simulink model "BLDCmotorControl_FOC_R2017b_fixdt"  (R2017b)
settings: Solver=FixedStepDiscrete  StartTime=0  StopTime=0.5  FixedStep=Ts  MaxStep=1e-6  RelTol=1e-6  AbsTol=1e-6  EnableMultiTasking=on
PreLoadFcn:
  | addpath(pwd);
  | addpath(genpath('01_Libraries'));
  | addpath(genpath('02_Figures'));
  | addpath(genpath('03_CreateParamTable'));
InitFcn:
  | init_model;
values from neighbouring files (symbols this model uses):
  a_elecAngle = 60    [init_model.m]
  b_diagEna = 1    [init_model.m]
  b_fieldWeakEna = 0    [init_model.m]
  b_selPhaABCurrMeas = 1    [init_model.m]
  cf_currFilt = 0.12    [init_model.m]
  cf_idKb = 1000 * Ts_ctrl    (= 0.06)    [init_model.m]
  cf_idKi = 100 * Ts_ctrl    (= 0.006)    [init_model.m]
  cf_idKp = 1    [init_model.m]
  cf_iqKb = 1000 * Ts_ctrl    (= 0.06)    [init_model.m]
  cf_iqKi = 100 * Ts_ctrl    (= 0.006)    [init_model.m]
  cf_iqKiLimProt = 40.7 * Ts_ctrl    (= 0.002442)    [init_model.m]
  cf_iqKp = 0.5    [init_model.m]
  cf_iqKpLimProt = 7.2    [init_model.m]
  cf_nKb = 1000 * Ts_ctrl    (= 0.06)    [init_model.m]
  cf_nKi = 20.4 * Ts_ctrl    (= 0.001224)    [init_model.m]
  cf_nKp = 1.18    [init_model.m]
  cf_nKpLimProt = 5    [init_model.m]
  cf_speedCoef = round(f_ctrl * a_mechAngle * (pi/180) * (30/pi))    [init_model.m]
  CTRL_COM = 0    [init_model.m]
  dV_openRate = 1000 * Ts_ctrl    (= 0.06)    [init_model.m]
  dz_cntTrnsDetHi = 40    [init_model.m]
  dz_cntTrnsDetLo = 20    [init_model.m]
  i_max = i_max * i_sca    (= 750)    [init_model.m]
  id_fieldWeak_M1 = [  0   0  0.05  0.25    1    2    3    4  4.5  4.8   5   5] * i_sca    [init_model.m]
  iq_max_M1 = sqrt(i_max^2 - iq_max_XA.^2)    [init_model.m]
  n_commAcvLo = 15    [init_model.m]
  n_commDeacvHi = 30    [init_model.m]
  n_max = 800    [init_model.m]
  n_stdStillDet = 3    [init_model.m]
  OPEN_MODE = 0    [init_model.m]
  r_cos_M1 = cos((a_elecAngle_XA + 30)*(pi/180))    [init_model.m]
  r_errInpTgtThres = 200    [init_model.m]
  r_sin_M1 = sin((a_elecAngle_XA + 30)*(pi/180))    [init_model.m]
  r_whl = 6.5 * 2.54 * 1e-2 / 2    (= 0.08255)    [init_model.m]
  SPD_MODE = 2    [init_model.m]
  t_errDequal = 2.0 * f_ctrl    (= 32000)    [init_model.m]
  t_errQual = 0.6 * f_ctrl    (= 9600)    [init_model.m]
  TRQ_MODE = 3    [init_model.m]
  Ts = 5e-6    (= 5e-06)    [init_model.m]
  Ts_ctrl = 6e-5    (= 6e-05)    [init_model.m]
  Vd_max = 1000 - V_margin    (= 900)    [init_model.m]
  vec_hallToPos = [0 2 0 1 4 3 5 0]    [init_model.m]
  VLT_MODE = 1    [init_model.m]
  Vq_max_M1 = sqrt(Vd_max^2 - Vq_max_XA.^2)    [init_model.m]
  z_commutMap_M1 = [-1 -1  0  1  1  0 ... (first row only)    [init_model.m]
  z_ctrlModReq = 1    [init_model.m]
  z_ctrlTypSel = 1    [init_model.m]
  z_maxCntRst = 2000    [init_model.m]
undefined symbols (not defined in the file or in its folder): DiscIntNeverNeededParam, sigbuilder_block, V_max, V_min
libraries: BLDC_controller_Lib x11, simulink x11, powerlib x6, pePwmGenerator x1
(part 3 of 3)

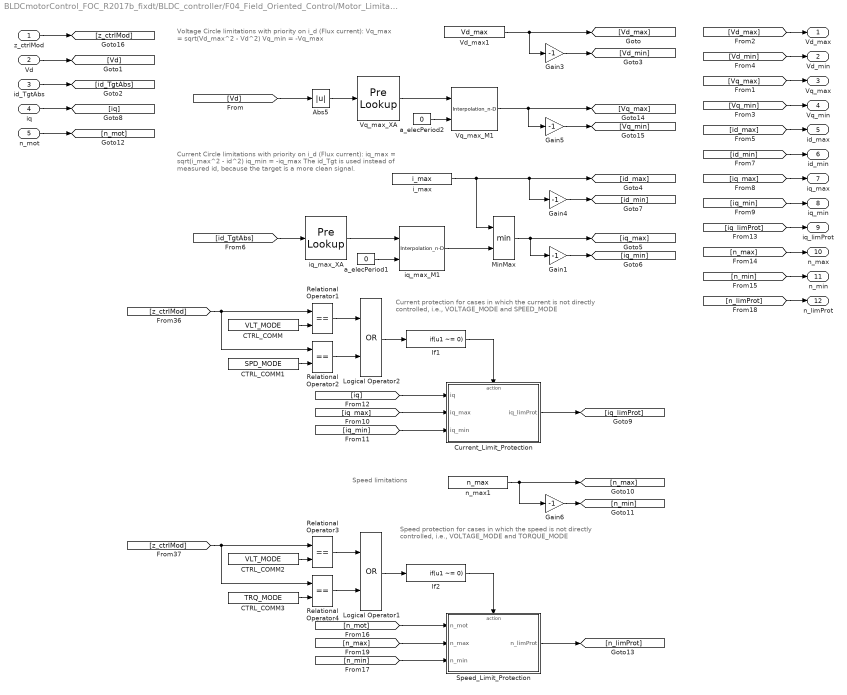
== system BLDCmotorControl_FOC_R2017b_fixdt/BLDC_controller/F04_Field_Oriented_Control/Motor_Limitations ==
  note: Voltage Circle limitations with priority on i_d (Flux current):
      | Vq_max = sqrt(Vd_max^2 - Vd^2)
      | Vq_min = -Vq_max
  note: Current Circle limitations with priority on i_d (Flux current):
      | iq_max = sqrt(i_max^2 - id^2)
      | iq_min = -iq_max
      |
      | The id_Tgt is used instead of measured id, because the target is a more clean signal.
  note: Speed limitations
  note: Current protection
      | for cases in which the current is not directly controlled, i.e., VOLTAGE_MODE and SPEED_MODE
  note: Speed protection
      | for cases in which the speed is not directly controlled, i.e., VOLTAGE_MODE and TORQUE_MODE
  z_ctrlMod : Inport
  Vd : Inport  Port=2
  id_TgtAbs : Inport  Port=3
  iq : Inport  Port=4
  n_mot : Inport  Port=5
  Abs5 : Abs  OutDataTypeStr=Inherit: Inherit via back propagation  RndMeth=Zero
  CTRL_COMM : Constant  Value=VLT_MODE  OutDataTypeStr=Inherit: Inherit via back propagation
  CTRL_COMM1 : Constant  Value=SPD_MODE  OutDataTypeStr=Inherit: Inherit via back propagation
  CTRL_COMM2 : Constant  Value=VLT_MODE  OutDataTypeStr=Inherit: Inherit via back propagation
  CTRL_COMM3 : Constant  Value=TRQ_MODE  OutDataTypeStr=Inherit: Inherit via back propagation
  Current_Limit_Protection : Subsystem
  Gain{1,3..6} (5 alike) : Gain  Tag=struct('comment',struct('text','','placement',1),'logdata',struct('maxnumvals',inf,'plotchannels',[],'loggingmode',3,'channels',1),'output',struct('variable','','description','','name','$S_$B','width',1,'address','','max',NaN,'min',NaN,'class','default','type','CONTINUOUS','scaling','','lsb',1,'offset',0,'arb',0,'freeze',1,'unit','','autoscalingmode',1,'lowerheadroom',1,'upperheadroom',1,'headroomunit','bit','keepdatatype',1,'checkmin',0,'checkmax',0,'castoutput',0,'show',0),'gain',struct('variable','','description','','name','$S_$B_gain','width',1,'address','','max',NaN,'min',NaN,'class','default','type','CONTINUOUS','scaling','','lsb',1,'offset',0,'arb',0,'freeze',1,'unit','','keepdatatype',1,'value','1','scalar',0,'tolerance',1),'scalingvalid',0,'date',730486)  Gain=-1  RndMeth=Zero  OutDataTypeStr=Inherit: Same as input  ParamDataTypeStr=Inherit: Same as input
  If1 : If  IfExpression=u1 ~= 0  ShowElse=off
  If2 : If  IfExpression=u1 ~= 0  ShowElse=off
  Logical Operator1 : Logic  Operator=OR  AllPortsSameDT=off  OutDataTypeStr=boolean
  Logical Operator2 : Logic  Operator=OR  AllPortsSameDT=off  OutDataTypeStr=boolean
  MinMax : MinMax  Inputs=2
  Relational Operator{1..4} (4 alike) : RelationalOperator  Operator===  OutDataTypeStr=boolean  RndMeth=Simplest
  Speed_Limit_Protection : Subsystem
  Vd_max1 : Constant  Value=Vd_max  OutDataTypeStr=fixdt(1,16,4)
  Vq_max_M1 : Interpolation_n-D  NumberOfTableDimensions=1  Table=Vq_max_M1  InterpMethod=Flat  ExtrapMethod=Clip  ValidIndexMayReachLast=on  OutDataTypeStr=fixdt(1,16,4)  InternalRulePriority=Speed  RndMeth=Simplest
      settings: InputPortMap=u0,u1
  Vq_max_XA : PreLookup  BreakpointsData=Vq_max_XA  OutputSelection=Index only  IndexSearchMethod=Evenly spaced points  BeginIndexSearchUsingPreviousIndexResult=on  IndexDataTypeStr=uint8  FractionDataTypeStr=fixdt(0,8,6)  RndMeth=Simplest
  a_elecPeriod1 : Constant  Value=0  OutDataTypeStr=uint8
  a_elecPeriod2 : Constant  Value=0  OutDataTypeStr=uint8
  i_max : Constant  Value=i_max  OutDataTypeStr=fixdt(1,16,4)
  iq_max_M1 : Interpolation_n-D  NumberOfTableDimensions=1  Table=iq_max_M1  InterpMethod=Flat  ExtrapMethod=Clip  ValidIndexMayReachLast=on  OutDataTypeStr=fixdt(1,16,4)  InternalRulePriority=Speed  RndMeth=Simplest
      settings: InputPortMap=u0,u1
  iq_max_XA : PreLookup  BreakpointsData=iq_max_XA  OutputSelection=Index only  IndexSearchMethod=Evenly spaced points  BeginIndexSearchUsingPreviousIndexResult=on  IndexDataTypeStr=uint8  FractionDataTypeStr=fixdt(0,8,6)  RndMeth=Simplest
  n_max1 : Constant  Value=n_max  OutDataTypeStr=fixdt(1,16,4)
  Vd_max : Outport  OutputWhenDisabled=reset  InitialOutput=V_max
  Vd_min : Outport  Port=2  OutputWhenDisabled=reset  InitialOutput=V_min
  Vq_max : Outport  Port=3  OutputWhenDisabled=reset  InitialOutput=V_max
  Vq_min : Outport  Port=4  OutputWhenDisabled=reset  InitialOutput=V_min
  id_max : Outport  Port=5  OutputWhenDisabled=reset  InitialOutput=V_max
  id_min : Outport  Port=6  OutputWhenDisabled=reset  InitialOutput=V_min
  iq_max : Outport  Port=7  OutputWhenDisabled=reset  InitialOutput=V_max
  iq_min : Outport  Port=8  OutputWhenDisabled=reset  InitialOutput=V_min
  iq_limProt : Outport  Port=9  OutputWhenDisabled=reset  InitialOutput=V_min
  n_max : Outport  Port=10  OutputWhenDisabled=reset  InitialOutput=V_max
  n_min : Outport  Port=11  OutputWhenDisabled=reset  InitialOutput=V_min
  n_limProt : Outport  Port=12  OutputWhenDisabled=reset  InitialOutput=V_min
  wires:
  Vq_max_XA/1 -> Vq_max_M1/1
  [Vq_min] -> Vq_min/1
  [Vq_max] -> Vq_max/1
  Gain5/1 -> [Vq_min]
  Vd_max1/1 -> Gain3/1, [Vd_max]
  [Vd] -> Abs5/1
  Vd/1 -> [Vd]
  id_TgtAbs/1 -> [id_TgtAbs]
  [Vd_max] -> Vd_max/1
  [Vd_min] -> Vd_min/1
  Gain3/1 -> [Vd_min]
  Gain4/1 -> [id_min]
  i_max/1 -> MinMax/1, Gain4/1, [id_max]
  [id_TgtAbs] -> iq_max_XA/1
  MinMax/1 -> [iq_max], Gain1/1
  Gain1/1 -> [iq_min]
  iq_max_XA/1 -> iq_max_M1/1
  [id_min] -> id_min/1
  [id_max] -> id_max/1
  [iq_max] -> iq_max/1
  [iq_min] -> iq_min/1
  iq/1 -> [iq]
  [iq_limProt] -> iq_limProt/1
  n_max1/1 -> [n_max], Gain6/1
  Gain6/1 -> [n_min]
  [n_min] -> n_min/1
  [n_max] -> n_max/1
  n_mot/1 -> [n_mot]
  [n_limProt] -> n_limProt/1
  z_ctrlMod/1 -> [z_ctrlMod]
  Relational Operator1/1 -> Logical Operator2/1
  [z_ctrlMod] -> Relational Operator2/1, Relational Operator1/1
  Logical Operator2/1 -> If1/1
  Relational Operator2/1 -> Logical Operator2/2
  CTRL_COMM/1 -> Relational Operator1/2
  CTRL_COMM1/1 -> Relational Operator2/2
  CTRL_COMM3/1 -> Relational Operator4/2
  CTRL_COMM2/1 -> Relational Operator3/2
  Relational Operator4/1 -> Logical Operator1/2
  Logical Operator1/1 -> If2/1
  [z_ctrlMod] -> Relational Operator3/1, Relational Operator4/1
  Relational Operator3/1 -> Logical Operator1/1
  [iq_max] -> Current_Limit_Protection/2(iq_max)
  [iq] -> Current_Limit_Protection/1(iq)
  [iq_min] -> Current_Limit_Protection/3(iq_min)
  Current_Limit_Protection/1(iq_limProt) -> [iq_limProt]
  [n_max] -> Speed_Limit_Protection/2(n_max)
  [n_mot] -> Speed_Limit_Protection/1(n_mot)
  [n_min] -> Speed_Limit_Protection/3(n_min)
  Speed_Limit_Protection/1(n_limProt) -> [n_limProt]
  If1/1 -> Current_Limit_Protection/Action
  If2/1 -> Speed_Limit_Protection/Action
  iq_max_M1/1 -> MinMax/2
  a_elecPeriod1/1 -> iq_max_M1/2
  Vq_max_M1/1 -> Gain5/1, [Vq_max]
  a_elecPeriod2/1 -> Vq_max_M1/2
  Abs5/1 -> Vq_max_XA/1

== system BLDCmotorControl_FOC_R2017b_fixdt/BLDC_controller/F04_Field_Oriented_Control/Open_Mode ==
  note: This will reduce the control command to 0 with a predefined rate.
  Vq_prev : Inport
  Action Port : ActionPort  InitializeStates=reset  ActionType=default
  Constant23 : Constant  Value=0  OutDataTypeStr=Inherit: Inherit via back propagation
  Data Type Conversion : DataTypeConversion  OutDataTypeStr=fixdt(1,28,16)
  Data Type Conversion1 : DataTypeConversion  OutDataTypeStr=fixdt(1,16,4)
  Gain3 : Gain  Tag=struct('comment',struct('text','','placement',1),'logdata',struct('maxnumvals',inf,'plotchannels',[],'loggingmode',3,'channels',1),'output',struct('variable','','description','','name','$S_$B','width',1,'address','','max',NaN,'min',NaN,'class','default','type','CONTINUOUS','scaling','','lsb',1,'offset',0,'arb',0,'freeze',1,'unit','','autoscalingmode',1,'lowerheadroom',1,'upperheadroom',1,'headroomunit','bit','keepdatatype',1,'checkmin',0,'checkmax',0,'castoutput',0,'show',0),'gain',struct('variable','','description','','name','$S_$B_gain','width',1,'address','','max',NaN,'min',NaN,'class','default','type','CONTINUOUS','scaling','','lsb',1,'offset',0,'arb',0,'freeze',1,'unit','','keepdatatype',1,'value','1','scalar',0,'tolerance',1),'scalingvalid',0,'date',730486)  Gain=-1  RndMeth=Zero  OutDataTypeStr=Inherit: Same as input
  Rate_Limiter : BLDC_controller_Lib/Rate_Limiter  SystemSampleTime=-1
  dV_openRate : Constant  Value=dV_openRate  OutDataTypeStr=fixdt(1,28,16)
  rising_edge_init : BLDC_controller_Lib/rising_edge_init
  Vq_Open : Outport
  wires:
  Vq_prev/1 -> [Vq_prev]
  Constant23/1 -> Rate_Limiter/1
  rising_edge_init/1 -> Rate_Limiter/3
  Gain3/1 -> Rate_Limiter/5
  dV_openRate/1 -> Gain3/1, Rate_Limiter/4
  Data Type Conversion1/1 -> [Vq_Open]
  [Vq_Open] -> Vq_Open/1
  Rate_Limiter/1 -> Data Type Conversion1/1
  [Vq_prev] -> Data Type Conversion/1
  Data Type Conversion/1 -> Rate_Limiter/2

== system BLDCmotorControl_FOC_R2017b_fixdt/BLDC_controller/F04_Field_Oriented_Control/Park_Transform ==
  note: Park Transform:
      | iq = -i_alpha*sin(angle) + i_beta*cos(angle)
      | id = i_alpha*cos(angle) + i_beta*sin(angle)
  i_apha : Inport
  i_beta : Inport  Port=2
  r_sin : Inport  Port=3
  r_cos : Inport  Port=4
  Divide{1..4} (4 alike) : Product  Inputs=**  RndMeth=Simplest  OutDataTypeStr=Inherit: Same as first input
  Sum1 : Sum  OutDataTypeStr=fixdt(1,16,4)  RndMeth=Simplest  SaturateOnIntegerOverflow=on
  Sum6 : Sum  Inputs=-+  OutDataTypeStr=fixdt(1,16,4)  RndMeth=Simplest  SaturateOnIntegerOverflow=on
  iq_Raw : Outport
  id_Raw : Outport  Port=2
  wires:
  r_sin/1 -> [r_sin]
  i_beta/1 -> [i_beta]
  i_apha/1 -> [i_apha]
  r_cos/1 -> [r_cos]
  [r_sin] -> Divide4/2
  [i_apha] -> Divide4/1
  Divide4/1 -> Sum6/1
  Divide1/1 -> Sum6/2
  [i_beta] -> Divide1/1
  [r_cos] -> Divide1/2
  Sum6/1 -> iq_Raw/1
  Divide2/1 -> Sum1/1
  [i_apha] -> Divide2/1
  [r_cos] -> Divide2/2
  Divide3/1 -> Sum1/2
  [i_beta] -> Divide3/1
  [r_sin] -> Divide3/2
  Sum1/1 -> id_Raw/1

== system BLDCmotorControl_FOC_R2017b_fixdt/BLDC_controller/F04_Field_Oriented_Control/Speed_Mode ==
  note: This product is necessary because the value is an input to the Integral part of the PI controller
  r_inpTgtSca : Inport
  Vq_max : Inport  Port=2
  Vq_min : Inport  Port=3
  n_mot : Inport  Port=4
  n_max : Inport  Port=5
  n_min : Inport  Port=6
  iq_limProt : Inport  Port=7
  Action Port : ActionPort  InitializeStates=reset  ActionType=case
  Divide1 : Product  Inputs=**  OutDataTypeStr=fixdt(1,16,10)  RndMeth=Simplest
  PI_backCalc_fixdt_n : BLDC_controller_Lib/PI_backCalc_fixdt  SystemSampleTime=-1
  Saturation Dynamic1 : simulink/Discontinuities/Saturation Dynamic  OutMin=[]  OutMax=[]  OutDataTypeStr=Inherit: Same as second input  OutDataType=fixdt(1, 16)  OutScaling=2^-10  DoSatur=off
  Signal Conversion2 : SignalConversion  OverrideOpt=off
  Sum3 : Sum  Inputs=|+-  RndMeth=Simplest  SaturateOnIntegerOverflow=on
  cf_iqKiLimProt : Constant  Value=cf_iqKiLimProt  OutDataTypeStr=fixdt(0,16,16)
  cf_nKb : Constant  Value=cf_nKb  OutDataTypeStr=fixdt(0,16,16)
  cf_nKi : Constant  Value=cf_nKi  VectorParams1D=off  OutDataTypeStr=fixdt(0,16,16)
  cf_nKp : Constant  Value=cf_nKp  OutDataTypeStr=fixdt(0,16,8)
  Vq_Spd : Outport
  wires:
  [Vq_min] -> PI_backCalc_fixdt_n/7
  [Vq_max] -> PI_backCalc_fixdt_n/6
  cf_nKi/1 -> PI_backCalc_fixdt_n/3
  cf_nKb/1 -> PI_backCalc_fixdt_n/4
  cf_nKp/1 -> PI_backCalc_fixdt_n/2
  [n_mot] -> Sum3/2
  Sum3/1 -> PI_backCalc_fixdt_n/1
  r_inpTgtSca/1 -> [r_inpTgtSca]
  Vq_max/1 -> [Vq_max]
  Vq_min/1 -> [Vq_min]
  n_mot/1 -> [n_mot]
  [n_min] -> Saturation Dynamic1/3
  [n_max] -> Saturation Dynamic1/1
  [r_inpTgtSca] -> Saturation Dynamic1/2
  Saturation Dynamic1/1 -> Sum3/1
  n_min/1 -> [n_min]
  n_max/1 -> [n_max]
  PI_backCalc_fixdt_n/1 -> Signal Conversion2/1
  iq_limProt/1 -> [iq_limProt]
  Divide1/1 -> PI_backCalc_fixdt_n/5
  cf_iqKiLimProt/1 -> Divide1/2
  [iq_limProt] -> Divide1/1
  Signal Conversion2/1 -> Vq_Spd/1

== system BLDCmotorControl_FOC_R2017b_fixdt/BLDC_controller/F04_Field_Oriented_Control/Torque_Mode ==
  r_inpTgtSca : Inport
  Vq_max : Inport  Port=2
  Vq_min : Inport  Port=3
  iq : Inport  Port=4
  iq_max : Inport  Port=5
  iq_min : Inport  Port=6
  n_limProt : Inport  Port=7
  Action Port : ActionPort  InitializeStates=reset  ActionType=case
  PI_backCalc_fixdt_Iq : BLDC_controller_Lib/PI_backCalc_fixdt  SystemSampleTime=-1
  Saturation Dynamic : simulink/Discontinuities/Saturation Dynamic  OutMin=[]  OutMax=[]  OutDataTypeStr=Inherit: Same as second input  OutDataType=fixdt(1, 16)  OutScaling=2^-10  DoSatur=off
  Signal Conversion2 : SignalConversion  OverrideOpt=off
  Sum1 : Sum  Inputs=|+-  RndMeth=Simplest  SaturateOnIntegerOverflow=on
  Sum2 : Sum  RndMeth=Simplest  SaturateOnIntegerOverflow=on
  cf_iqKb : Constant  Value=cf_iqKb  OutDataTypeStr=fixdt(0,16,16)
  cf_iqKi : Constant  Value=cf_iqKi  OutDataTypeStr=fixdt(0,16,16)
  cf_iqKp : Constant  Value=cf_iqKp  OutDataTypeStr=fixdt(0,16,8)
  constant : Constant  Value=0  OutDataTypeStr=Inherit: Inherit via back propagation
  Vq_Trq : Outport
  wires:
  cf_iqKi/1 -> PI_backCalc_fixdt_Iq/3
  [r_inpTgtSca] -> Sum2/1
  [Vq_max] -> PI_backCalc_fixdt_Iq/6
  [Vq_min] -> PI_backCalc_fixdt_Iq/7
  [iq] -> Sum1/2
  Sum1/1 -> PI_backCalc_fixdt_Iq/1
  cf_iqKb/1 -> PI_backCalc_fixdt_Iq/4
  cf_iqKp/1 -> PI_backCalc_fixdt_Iq/2
  Vq_max/1 -> [Vq_max]
  r_inpTgtSca/1 -> [r_inpTgtSca]
  Vq_min/1 -> [Vq_min]
  iq/1 -> [iq]
  PI_backCalc_fixdt_Iq/1 -> Signal Conversion2/1
  iq_min/1 -> [iq_min]
  iq_max/1 -> [iq_max]
  [iq_min] -> Saturation Dynamic/3
  [iq_max] -> Saturation Dynamic/1
  Sum2/1 -> Saturation Dynamic/2
  [n_limProt] -> Sum2/2
  n_limProt/1 -> [n_limProt]
  constant/1 -> PI_backCalc_fixdt_Iq/5
  Signal Conversion2/1 -> Vq_Trq/1
  Saturation Dynamic/1 -> Sum1/1

== system BLDCmotorControl_FOC_R2017b_fixdt/BLDC_controller/F04_Field_Oriented_Control/Vd_Calculation ==
  id_Tgt : Inport
  id : Inport  Port=2
  Vd_max : Inport  Port=3
  Vd_min : Inport  Port=4
  id_max : Inport  Port=5
  id_min : Inport  Port=6
  Action Port : ActionPort  InitializeStates=reset  ActionType=then
  PI_backCalc_fixdt_Id : BLDC_controller_Lib/PI_backCalc_fixdt  SystemSampleTime=-1
  Saturation Dynamic : simulink/Discontinuities/Saturation Dynamic  OutMin=[]  OutMax=[]  OutDataTypeStr=Inherit: Same as second input  OutDataType=fixdt(1, 16)  OutScaling=2^-10  DoSatur=off
  Sum3 : Sum  Inputs=|+-  RndMeth=Simplest  SaturateOnIntegerOverflow=on
  cf_idKb : Constant  Value=cf_idKb  OutDataTypeStr=fixdt(0,16,16)
  cf_idKi : Constant  Value=cf_idKi  OutDataTypeStr=fixdt(0,16,16)
  cf_idKp : Constant  Value=cf_idKp  OutDataTypeStr=fixdt(0,16,8)
  constant : Constant  Value=0  OutDataTypeStr=Inherit: Inherit via back propagation
  Vd : Outport  OutputWhenDisabled=reset  InitialOutput=0
  wires:
  [id] -> Sum3/2
  [id_Tgt] -> Saturation Dynamic/2
  id_Tgt/1 -> [id_Tgt]
  id/1 -> [id]
  Vd_min/1 -> [Vd_min]
  Vd_max/1 -> [Vd_max]
  id_max/1 -> [id_max]
  id_min/1 -> [id_min]
  Saturation Dynamic/1 -> Sum3/1
  [id_max] -> Saturation Dynamic/1
  [id_min] -> Saturation Dynamic/3
  Sum3/1 -> PI_backCalc_fixdt_Id/1
  [Vd_max] -> PI_backCalc_fixdt_Id/6
  [Vd_min] -> PI_backCalc_fixdt_Id/7
  cf_idKp/1 -> PI_backCalc_fixdt_Id/2
  cf_idKi/1 -> PI_backCalc_fixdt_Id/3
  cf_idKb/1 -> PI_backCalc_fixdt_Id/4
  constant/1 -> PI_backCalc_fixdt_Id/5
  PI_backCalc_fixdt_Id/1 -> Vd/1

== system BLDCmotorControl_FOC_R2017b_fixdt/BLDC_controller/F04_Field_Oriented_Control/Voltage_Mode ==
  r_inpTgtSca : Inport
  Vq_max : Inport  Port=2
  Vq_min : Inport  Port=3
  iq_limProt : Inport  Port=4
  n_limProt : Inport  Port=5
  Action Port : ActionPort  InitializeStates=reset  ActionType=case
  Saturation Dynamic1 : simulink/Discontinuities/Saturation Dynamic  OutMin=[]  OutMax=[]  OutDataTypeStr=Inherit: Same as second input  OutDataType=fixdt(1, 16)  OutScaling=2^-10  DoSatur=off
  Signal Conversion2 : SignalConversion  OverrideOpt=off
  Sum3 : Sum  Inputs=+++  RndMeth=Simplest  SaturateOnIntegerOverflow=on
  Vq_Vlt : Outport
  wires:
  r_inpTgtSca/1 -> [r_inpTgtSca]
  [Vq_min] -> Saturation Dynamic1/3
  [Vq_max] -> Saturation Dynamic1/1
  Vq_max/1 -> [Vq_max]
  Vq_min/1 -> [Vq_min]
  iq_limProt/1 -> [iq_limProt]
  n_limProt/1 -> [n_limProt]
  Sum3/1 -> Saturation Dynamic1/2
  [r_inpTgtSca] -> Sum3/1
  Signal Conversion2/1 -> Vq_Vlt/1
  [iq_limProt] -> Sum3/2
  [n_limProt] -> Sum3/3
  Saturation Dynamic1/1 -> Signal Conversion2/1

== system BLDCmotorControl_FOC_R2017b_fixdt/PWM_gates/PWM_generator1/__InputSSForSFun__ ==
  DC : Inport  SampleTime=Ts
  __UniqueOutportName__1__ : Outport
  wires:
  DC/1 -> __UniqueOutportName__1__/1

== system BLDCmotorControl_FOC_R2017b_fixdt/PWM_gates/PWM_generator1/__OutputSSForSFun__ ==
  __UniqueInportName__1__ : Inport
  PWM : Outport
  wires:
  __UniqueInportName__1__/1 -> PWM/1

== system BLDCmotorControl_FOC_R2017b_fixdt/PWM_gates/PWM_generator12/__InputSSForSFun__ ==
  DC : Inport  SampleTime=Ts
  __UniqueOutportName__1__ : Outport
  wires:
  DC/1 -> __UniqueOutportName__1__/1

== system BLDCmotorControl_FOC_R2017b_fixdt/PWM_gates/PWM_generator12/__OutputSSForSFun__ ==
  __UniqueInportName__1__ : Inport
  PWM : Outport
  wires:
  __UniqueInportName__1__/1 -> PWM/1

== system BLDCmotorControl_FOC_R2017b_fixdt/PWM_gates/PWM_generator2/__InputSSForSFun__ ==
  DC : Inport  SampleTime=Ts
  __UniqueOutportName__1__ : Outport
  wires:
  DC/1 -> __UniqueOutportName__1__/1

== system BLDCmotorControl_FOC_R2017b_fixdt/PWM_gates/PWM_generator2/__OutputSSForSFun__ ==
  __UniqueInportName__1__ : Inport
  PWM : Outport
  wires:
  __UniqueInportName__1__/1 -> PWM/1

== system BLDCmotorControl_FOC_R2017b_fixdt/PWM_gates/PWM_generator3/__InputSSForSFun__ ==
  DC : Inport  SampleTime=Ts
  __UniqueOutportName__1__ : Outport
  wires:
  DC/1 -> __UniqueOutportName__1__/1

== system BLDCmotorControl_FOC_R2017b_fixdt/PWM_gates/PWM_generator3/__OutputSSForSFun__ ==
  __UniqueInportName__1__ : Inport
  PWM : Outport
  wires:
  __UniqueInportName__1__/1 -> PWM/1

== system BLDCmotorControl_FOC_R2017b_fixdt/PWM_gates/PWM_generator4/__InputSSForSFun__ ==
  DC : Inport  SampleTime=Ts
  __UniqueOutportName__1__ : Outport
  wires:
  DC/1 -> __UniqueOutportName__1__/1

== system BLDCmotorControl_FOC_R2017b_fixdt/PWM_gates/PWM_generator4/__OutputSSForSFun__ ==
  __UniqueInportName__1__ : Inport
  PWM : Outport
  wires:
  __UniqueInportName__1__/1 -> PWM/1

== system BLDCmotorControl_FOC_R2017b_fixdt/PWM_gates/PWM_generator5/__InputSSForSFun__ ==
  DC : Inport  SampleTime=Ts
  __UniqueOutportName__1__ : Outport
  wires:
  DC/1 -> __UniqueOutportName__1__/1

== system BLDCmotorControl_FOC_R2017b_fixdt/PWM_gates/PWM_generator5/__OutputSSForSFun__ ==
  __UniqueInportName__1__ : Inport
  PWM : Outport
  wires:
  __UniqueInportName__1__/1 -> PWM/1

== system BLDCmotorControl_FOC_R2017b_fixdt/BLDC_controller/F01_Estimations/F01_01_Input_Scaling/Commutation_Control_Type ==
  r_inpTgt : Inport
  Action Port : ActionPort  InitializeStates=reset  ActionType=then
  r_inpTgtScaCOM : Outport
  wires:
  r_inpTgt/1 -> r_inpTgtScaCOM/1

== system BLDCmotorControl_FOC_R2017b_fixdt/BLDC_controller/F01_Estimations/F01_01_Input_Scaling/FOC_Control_Type ==
  r_inpTgt : Inport
  z_ctrlModPrev : Inport  Port=2
  Action Port : ActionPort  InitializeStates=reset  ActionType=else
  Divide1 : Product  Inputs=**  OutDataTypeStr=fixdt(1,16,4)  RndMeth=Simplest
  Divide4 : Product  Inputs=*/  OutDataTypeStr=fixdt(0,16,12)  RndMeth=Simplest
  Mux : Mux
  Selector : Selector  IndexMode=Zero-based  InputPortWidth=4  IndexOptions=Index vector (port)  Indices=[1 3]  OutputSizes=1
  Vd_max : Constant  Value=Vd_max  OutDataTypeStr=fixdt(1,16,4)
  constant : Constant  Value=1000  OutDataTypeStr=Inherit: Inherit via back propagation
  constant1 : Constant  Value=0  OutDataTypeStr=Inherit: Inherit via back propagation
  i_max : Constant  Value=i_max  OutDataTypeStr=fixdt(1,16,4)
  n_max : Constant  Value=n_max  OutDataTypeStr=fixdt(1,16,4)
  r_inpTgtScaFOC : Outport
  wires:
  r_inpTgt/1 -> [r_inpTgt]
  [r_inpTgtScaFOC] -> r_inpTgtScaFOC/1
  z_ctrlModPrev/1 -> [z_ctrlModPrev]
  constant/1 -> Divide4/2
  Selector/1 -> Divide4/1
  constant1/1 -> Mux/1
  i_max/1 -> Mux/4
  Vd_max/1 -> Mux/2
  Mux/1 -> Selector/1
  n_max/1 -> Mux/3
  [z_ctrlModPrev] -> Selector/2
  Divide4/1 -> Divide1/2
  Divide1/1 -> [r_inpTgtScaFOC]
  [r_inpTgt] -> Divide1/1

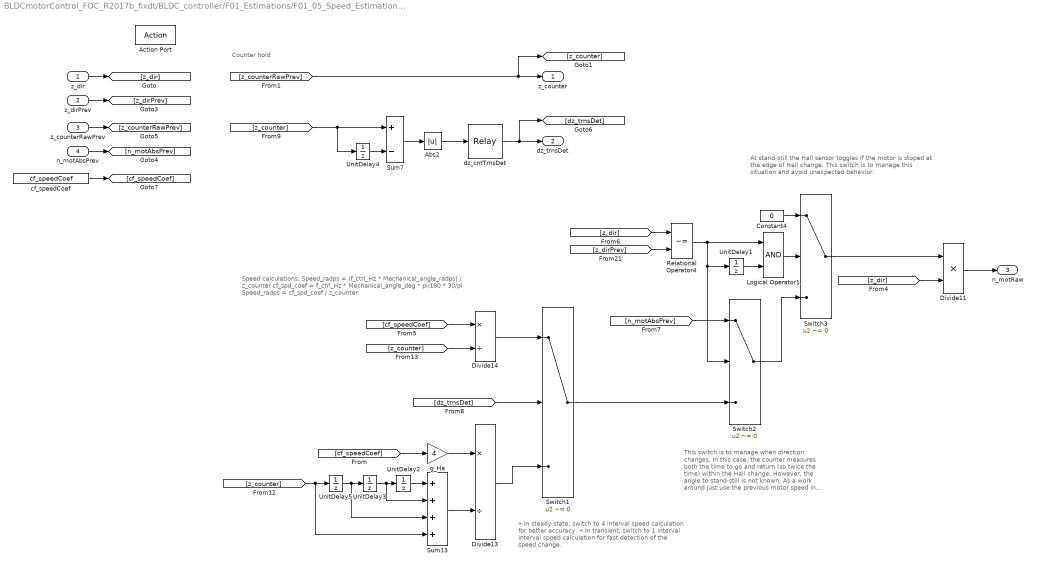
== system BLDCmotorControl_FOC_R2017b_fixdt/BLDC_controller/F01_Estimations/F01_05_Speed_Estimation/Raw_Motor_Speed_Estimation ==
  note: Speed calculations:
      | Speed_radps = (f_ctrl_Hz * Mechanical_angle_radps) / z_counter
      | cf_spd_coef = f_ctrl_Hz * Mechanical_angle_deg * pi/180 * 30/pi
      | Speed_radps = cf_spd_coef / z_counter
  note: Counter hold
  note: • In steady state, switch to 4 interval speed calculation for better accuracy.
      | • In transient, switch to 1 interval interval spped calculation for fast detection of the speed change.
  note: This switch is to manage when direction changes. In this case, the counter measures both the time to go and return (so twice the time) within the Hall change. However, the angle to stand-still is not known. As a work around just use the previous motor speed in absolute value.
  note: At stand-still the Hall sensor toggles if the motor is stoped at the edge of Hall change. This switch is to manage this situation and avoid unexpected behavior.
  z_dir : Inport
  z_dirPrev : Inport  Port=2
  z_counterRawPrev : Inport  Port=3
  n_motAbsPrev : Inport  Port=4
  Action Port : ActionPort  ActionType=then
  Abs2 : Abs  OutDataTypeStr=Inherit: Inherit via back propagation  RndMeth=Zero
  Constant4 : Constant  Value=0  OutDataTypeStr=Inherit: Inherit via back propagation
  Divide11 : Product  Inputs=**  RndMeth=Simplest  OutDataTypeStr=Inherit: Same as first input
  Divide13 : Product  Inputs=*/  OutDataTypeStr=fixdt(1,16,4)  RndMeth=Simplest
  Divide14 : Product  Inputs=*/  OutDataTypeStr=fixdt(1,16,4)  RndMeth=Simplest
  Logical Operator1 : Logic  AllPortsSameDT=off  OutDataTypeStr=boolean
  Relational Operator4 : RelationalOperator  Operator=~=  OutDataTypeStr=boolean  RndMeth=Simplest
  Sum13 : Sum  Inputs=++++  RndMeth=Simplest  InputSameDT=on  OutDataTypeStr=Inherit: Same as first input
  Sum7 : Sum  Inputs=+-  RndMeth=Simplest  InputSameDT=on  OutDataTypeStr=Inherit: Same as first input
  Switch1 : Switch  Tag=struct('comment',struct('text','','placement',1),'logdata',struct('maxnumvals',inf,'plotchannels',[],'loggingmode',3,'channels',1),'output',struct('variable','','description','','name','$S_$B','width',1,'address','','max',NaN,'min',NaN,'class','default','type','CONTINUOUS','scaling','','lsb',1,'offset',0,'arb',0,'freeze',1,'unit','','autoscalingmode',1,'lowerheadroom',1,'upperheadroom',1,'headroomunit','bit','keepdatatype',1,'checkmin',0,'checkmax',0,'castoutput',0,'show',0),'threshold',struct('variable','','description','','name','$S_$B_threshold','width',1,'address','','max',NaN,'min',NaN,'class','default','type','CONTINUOUS','scaling','','lsb',1,'offset',0,'arb',0,'freeze',1,'unit','','keepdatatype',1,'value','0','scalar',0,'criteria',3),'scalingvalid',0,'date',733087.49614628474,'inheritscaling',0)  Criteria=u2 ~= 0  InputSameDT=on
      settings: AttributesFormatString=threshold=%<threshold>\nCriteria : %<Criteria>
  Switch2 : Switch  Tag=struct('comment',struct('text','','placement',1),'logdata',struct('maxnumvals',inf,'plotchannels',[],'loggingmode',3,'channels',1),'output',struct('variable','','description','','name','$S_$B','width',1,'address','','max',NaN,'min',NaN,'class','default','type','CONTINUOUS','scaling','','lsb',1,'offset',0,'arb',0,'freeze',1,'unit','','autoscalingmode',1,'lowerheadroom',1,'upperheadroom',1,'headroomunit','bit','keepdatatype',1,'checkmin',0,'checkmax',0,'castoutput',0,'show',0),'threshold',struct('variable','','description','','name','$S_$B_threshold','width',1,'address','','max',NaN,'min',NaN,'class','default','type','CONTINUOUS','scaling','','lsb',1,'offset',0,'arb',0,'freeze',1,'unit','','keepdatatype',1,'value','0','scalar',0,'criteria',3),'scalingvalid',0,'date',733087.49614628474,'inheritscaling',0)  Criteria=u2 ~= 0  InputSameDT=on
      settings: AttributesFormatString=threshold=%<threshold>\nCriteria : %<Criteria>
  Switch3 : Switch  Tag=struct('comment',struct('text','','placement',1),'logdata',struct('maxnumvals',inf,'plotchannels',[],'loggingmode',3,'channels',1),'output',struct('variable','','description','','name','$S_$B','width',1,'address','','max',NaN,'min',NaN,'class','default','type','CONTINUOUS','scaling','','lsb',1,'offset',0,'arb',0,'freeze',1,'unit','','autoscalingmode',1,'lowerheadroom',1,'upperheadroom',1,'headroomunit','bit','keepdatatype',1,'checkmin',0,'checkmax',0,'castoutput',0,'show',0),'threshold',struct('variable','','description','','name','$S_$B_threshold','width',1,'address','','max',NaN,'min',NaN,'class','default','type','CONTINUOUS','scaling','','lsb',1,'offset',0,'arb',0,'freeze',1,'unit','','keepdatatype',1,'value','0','scalar',0,'criteria',3),'scalingvalid',0,'date',733087.49614628474,'inheritscaling',0)  Criteria=u2 ~= 0  InputSameDT=on
      settings: AttributesFormatString=threshold=%<threshold>\nCriteria : %<Criteria>
  UnitDelay{1..5} (5 alike) : UnitDelay  SampleTime=-1
      settings: AttributesFormatString=Ini=%<X0>
  cf_speedCoef : Constant  Value=cf_speedCoef  OutDataTypeStr=fixdt(0,16,0)
  dz_cntTrnsDet : Relay  OnSwitchValue=dz_cntTrnsDetHi  OffSwitchValue=dz_cntTrnsDetLo  OutDataTypeStr=boolean
  g_Ha : Gain  Gain=4  OutDataTypeStr=Inherit: Inherit via back propagation  RndMeth=Zero  ParamDataTypeStr=Inherit: Same as input
  z_counter : Outport  InitialOutput=z_maxCntRst
  dz_trnsDet : Outport  Port=2
  n_motRaw : Outport  Port=3
  wires:
  z_dir/1 -> [z_dir]
  z_dirPrev/1 -> [z_dirPrev]
  z_counterRawPrev/1 -> [z_counterRawPrev]
  [z_dir] -> Divide11/2
  UnitDelay3/1 -> UnitDelay2/1, Sum13/2
  UnitDelay5/1 -> UnitDelay3/1, Sum13/3
  [z_counter] -> UnitDelay5/1, Sum13/4
  [cf_speedCoef] -> g_Ha/1
  Sum13/1 -> Divide13/2
  g_Ha/1 -> Divide13/1
  [z_counter] -> Divide14/2
  [cf_speedCoef] -> Divide14/1
  UnitDelay4/1 -> Sum7/2
  [z_counter] -> UnitDelay4/1, Sum7/1
  Sum7/1 -> Abs2/1
  Abs2/1 -> dz_cntTrnsDet/1
  cf_speedCoef/1 -> [cf_speedCoef]
  UnitDelay2/1 -> Sum13/1
  [z_dir] -> Relational Operator4/1
  [z_dirPrev] -> Relational Operator4/2
  UnitDelay1/1 -> Logical Operator1/2
  Relational Operator4/1 -> UnitDelay1/1, Switch2/2, Logical Operator1/1
  Logical Operator1/1 -> Switch3/2
  Switch2/1 -> Switch3/3
  Constant4/1 -> Switch3/1
  Switch3/1 -> Divide11/1
  n_motAbsPrev/1 -> [n_motAbsPrev]
  [n_motAbsPrev] -> Switch2/1
  [z_counterRawPrev] -> z_counter/1, [z_counter]
  dz_cntTrnsDet/1 -> [dz_trnsDet], dz_trnsDet/1
  Divide13/1 -> Switch1/3
  Divide11/1 -> n_motRaw/1
  [dz_trnsDet] -> Switch1/2
  Switch1/1 -> Switch2/3
  Divide14/1 -> Switch1/1

== system BLDCmotorControl_FOC_R2017b_fixdt/BLDC_controller/F04_Field_Oriented_Control/Clarke_Transform/Clarke_PhasesAB ==
  note: Clarke Transform:
      | i_alpha = i_phaA
      | i_beta = ((1/sqrt(3))*i_phaA + (2/sqrt(3))*i_phaB)
  i_phaA : Inport
  i_phaB : Inport  Port=2
  Action Port : ActionPort  ActionType=then
  Gain2 : Gain  Tag=struct('comment',struct('text','','placement',1),'logdata',struct('maxnumvals',inf,'plotchannels',[],'loggingmode',3,'channels',1),'output',struct('variable','','description','','name','$S_$B','width',1,'address','','max',NaN,'min',NaN,'class','default','type','CONTINUOUS','scaling','','lsb',1,'offset',0,'arb',0,'freeze',1,'unit','','autoscalingmode',1,'lowerheadroom',1,'upperheadroom',1,'headroomunit','bit','keepdatatype',1,'checkmin',0,'checkmax',0,'castoutput',0,'show',0),'gain',struct('variable','','description','','name','$S_$B_gain','width',1,'address','','max',NaN,'min',NaN,'class','default','type','CONTINUOUS','scaling','','lsb',1,'offset',0,'arb',0,'freeze',1,'unit','','keepdatatype',1,'value','1','scalar',0,'tolerance',1),'scalingvalid',0,'date',730486)  Gain=2/sqrt(3)  RndMeth=Zero  OutDataTypeStr=Inherit: Same as input
  Gain4 : Gain  Tag=struct('comment',struct('text','','placement',1),'logdata',struct('maxnumvals',inf,'plotchannels',[],'loggingmode',3,'channels',1),'output',struct('variable','','description','','name','$S_$B','width',1,'address','','max',NaN,'min',NaN,'class','default','type','CONTINUOUS','scaling','','lsb',1,'offset',0,'arb',0,'freeze',1,'unit','','autoscalingmode',1,'lowerheadroom',1,'upperheadroom',1,'headroomunit','bit','keepdatatype',1,'checkmin',0,'checkmax',0,'castoutput',0,'show',0),'gain',struct('variable','','description','','name','$S_$B_gain','width',1,'address','','max',NaN,'min',NaN,'class','default','type','CONTINUOUS','scaling','','lsb',1,'offset',0,'arb',0,'freeze',1,'unit','','keepdatatype',1,'value','1','scalar',0,'tolerance',1),'scalingvalid',0,'date',730486)  Gain=1/sqrt(3)  RndMeth=Zero  OutDataTypeStr=Inherit: Same as input
  Signal Conversion2 : SignalConversion  OverrideOpt=off
  Sum1 : Sum  OutDataTypeStr=fixdt(1,16,4)  RndMeth=Simplest  SaturateOnIntegerOverflow=on
  i_alphaAB : Outport
  i_betaAB : Outport  Port=2
  wires:
  i_phaB/1 -> [i_phaB]
  i_phaA/1 -> [i_phaA]
  [i_phaA] -> Signal Conversion2/1, Gain4/1
  Gain2/1 -> Sum1/2
  [i_phaB] -> Gain2/1
  Gain4/1 -> Sum1/1
  Sum1/1 -> i_betaAB/1
  Signal Conversion2/1 -> i_alphaAB/1

== system BLDCmotorControl_FOC_R2017b_fixdt/BLDC_controller/F04_Field_Oriented_Control/Clarke_Transform/Clarke_PhasesBC ==
  note: Clarke Transform:
      | i_alpha = - i_phaB - i_phaC
      | i_beta = (1/sqrt(3)) * (i_phaB - i_phaC)
  i_phaB : Inport
  i_phaC : Inport  Port=2
  Action Port : ActionPort  ActionType=else
  Gain2 : Gain  Tag=struct('comment',struct('text','','placement',1),'logdata',struct('maxnumvals',inf,'plotchannels',[],'loggingmode',3,'channels',1),'output',struct('variable','','description','','name','$S_$B','width',1,'address','','max',NaN,'min',NaN,'class','default','type','CONTINUOUS','scaling','','lsb',1,'offset',0,'arb',0,'freeze',1,'unit','','autoscalingmode',1,'lowerheadroom',1,'upperheadroom',1,'headroomunit','bit','keepdatatype',1,'checkmin',0,'checkmax',0,'castoutput',0,'show',0),'gain',struct('variable','','description','','name','$S_$B_gain','width',1,'address','','max',NaN,'min',NaN,'class','default','type','CONTINUOUS','scaling','','lsb',1,'offset',0,'arb',0,'freeze',1,'unit','','keepdatatype',1,'value','1','scalar',0,'tolerance',1),'scalingvalid',0,'date',730486)  Gain=1/sqrt(3)  RndMeth=Zero  OutDataTypeStr=Inherit: Same as input
  Sum1 : Sum  Inputs=--  OutDataTypeStr=fixdt(1,16,4)  RndMeth=Simplest  SaturateOnIntegerOverflow=on
  Sum3 : Sum  Inputs=+-  OutDataTypeStr=fixdt(1,16,4)  RndMeth=Simplest  SaturateOnIntegerOverflow=on
  i_alphaBC : Outport
  i_betaBC : Outport  Port=2
  wires:
  [i_phaC] -> Sum1/2
  [i_phaB] -> Sum1/1
  [i_phaC] -> Sum3/2
  Gain2/1 -> i_betaBC/1
  Sum3/1 -> Gain2/1
  [i_phaB] -> Sum3/1
  Sum1/1 -> i_alphaBC/1
  i_phaB/1 -> [i_phaB]
  i_phaC/1 -> [i_phaC]

== system BLDCmotorControl_FOC_R2017b_fixdt/BLDC_controller/F04_Field_Oriented_Control/Motor_Limitations/Current_Limit_Protection ==
  iq : Inport
  iq_max : Inport  Port=2
  iq_min : Inport  Port=3
  Action Port : ActionPort  InitializeStates=reset  ActionType=then
  Divide4 : Product  Inputs=**  RndMeth=Simplest  SaturateOnIntegerOverflow=on  OutDataTypeStr=Inherit: Same as first input
  Saturation Dynamic : simulink/Discontinuities/Saturation Dynamic  OutMin=[]  OutMax=[]  OutDataTypeStr=Inherit: Same as second input  OutDataType=fixdt(1, 16)  OutScaling=2^-10  DoSatur=off
  Sum3 : Sum  Inputs=|+-  RndMeth=Simplest
  cf_iqKpLimProt : Constant  Value=cf_iqKpLimProt  OutDataTypeStr=fixdt(0,16,6)
  iq_limProt : Outport  OutputWhenDisabled=reset  InitialOutput=0
  wires:
  Sum3/1 -> Divide4/1
  iq/1 -> Sum3/2, Saturation Dynamic/2
  cf_iqKpLimProt/1 -> Divide4/2
  Saturation Dynamic/1 -> Sum3/1
  iq_max/1 -> Saturation Dynamic/1
  iq_min/1 -> Saturation Dynamic/3
  Divide4/1 -> iq_limProt/1

== system BLDCmotorControl_FOC_R2017b_fixdt/BLDC_controller/F04_Field_Oriented_Control/Motor_Limitations/Speed_Limit_Protection ==
  n_mot : Inport
  n_max : Inport  Port=2
  n_min : Inport  Port=3
  Action Port : ActionPort  InitializeStates=reset  ActionType=then
  Divide1 : Product  Inputs=**  RndMeth=Simplest  SaturateOnIntegerOverflow=on  OutDataTypeStr=Inherit: Same as first input
  Saturation Dynamic1 : simulink/Discontinuities/Saturation Dynamic  OutMin=[]  OutMax=[]  OutDataTypeStr=Inherit: Same as second input  OutDataType=fixdt(1, 16)  OutScaling=2^-10  DoSatur=off
  Sum1 : Sum  Inputs=|+-  RndMeth=Simplest
  cf_nKpLimProt : Constant  Value=cf_nKpLimProt  OutDataTypeStr=fixdt(0,16,6)
  n_limProt : Outport  OutputWhenDisabled=reset  InitialOutput=0
  wires:
  Saturation Dynamic1/1 -> Sum1/1
  n_min/1 -> Saturation Dynamic1/3
  Sum1/1 -> Divide1/1
  n_max/1 -> Saturation Dynamic1/1
  cf_nKpLimProt/1 -> Divide1/2
  n_mot/1 -> Sum1/2, Saturation Dynamic1/2
  Divide1/1 -> n_limProt/1

== stateflow chart BLDCmotorControl_FOC_R2017b_fixdt/BLDC_controller/F03_Control_Mode_Manager/F02_02_Control_Mode_Manager ==
  state OPEN
    entry:
    z_ctrlMod = OPEN_MODE;
  state ACTIVE
    state TORQUE_MODE
      entry:
      z_ctrlMod = TRQ_MODE;
    state SPEED_MODE
      entry:
      z_ctrlMod = SPD_MODE;
    state VOLTAGE_MODE
      entry:
      z_ctrlMod = VLT_MODE;
    (default) -> (junction 7)
    (junction 7) -> TORQUE_MODE [order 1] : [b_toTrqMod]
    (junction 7) -> (junction 8) [order 2]
    (junction 8) -> SPEED_MODE [order 1] : [b_toSpdMod]
    (junction 8) -> (junction 29) [order 2]
    (junction 29) -> VOLTAGE_MODE
  (default) -> OPEN
  OPEN -> ACTIVE : [b_toActive]
  ACTIVE -> OPEN : [b_toOpen]
  data: b_toOpen input boolean; b_toActive input boolean; b_toSpdMod input boolean; z_ctrlMod output uint8; OPEN_MODE constant uint8 =OPEN_MODE; TRQ_MODE constant uint8 =TRQ_MODE; SPD_MODE constant uint8 =SPD_MODE; VLT_MODE constant uint8 =VLT_MODE; b_toTrqMod input boolean
